simulink model "Racing_2019"  (R2017a)
settings: Solver=FixedStepDiscrete  StartTime=0.0  StopTime=Inf  FixedStep=1e-3  RelTol=1e-3  EnableMultiTasking=on
PostLoadFcn:
  | , if any(exist('dsrtsu_mdlpostloadfcn', 'file') == [2, 3, 6]), try dsrtsu_mdlpostloadfcn('Execute', bdroot); catch fprintf('Error in PostLoadFcn (dsrtsu_mdlpostloadfcn) for model "%s":\n %s\n', bdroot, lasterr); end, end,
undefined symbols (not defined in the file): Accu_Fans_Enable, Accu_Fans_ON, Accu_Fans_PWM, APPS_Bypass, APPS_Value, AUX_Error_Time, Batt_Temp_High_Threshold, Batt_Temp_Low_Threshold, BMS_Error_Time, BMS_Reset, BMS_Reset_Enable, BMS_Status_Bypass, Brake_Plausibility_Threshold, Brake_Threshold, Brakelight_Test, Braking_Torque, BSPD_State_Bypass, Buzzer, Buzzer_Silent, Buzzer_Test, Calibrate, CAN_Rx_FMEA_Enable, CAN_Status_FMEA_Enable, CAN_Tx_FMEA_Enable, Car_Reset, Car_Reset_Enable, Dash_Fan_PWM, DiscIntNeverNeededParam, DRS_Enable, DRS_PWM_OFF, DRS_PWM_ON, ED_Enable, ED_On, Eject_USB, Enable_Kill, Enable_LED_Test, Fans_Left_Enable, Fans_Left_ON, Fans_Left_PWM, Fans_Right_Enable, Fans_Right_ON, Fans_Right_PWM, I_MAX, IGBT_Temp_High_Threshold, IGBT_Temp_Low_Threshold, Inverter_CAN_Tx_Enable, Inverter_Frequency, KW_Max_Regen_Reset, KW_Max_Reset, LV_DCDC_Temp_High_Threshold, LV_DCDC_Temp_Low_Threshold, magnitude, Plausibility_Bypass, Power_Limiter_Killswitch, Power_Target_kW, Pump_Left_Enable, Pump_Left_ON, Pump_Right_Enable, Pump_Right_ON, Pump_Signal_Left ... (+13)
libraries: rtiusbflightreclib x206, simulink x153, rtican x52, powerlib_meascontrol x47, simulink_extras x17, rti1401lib_adc_type4 x6, rti1401lib_dio_type4 x3, rti1401lib_II_base x1
(part 6 of 23)

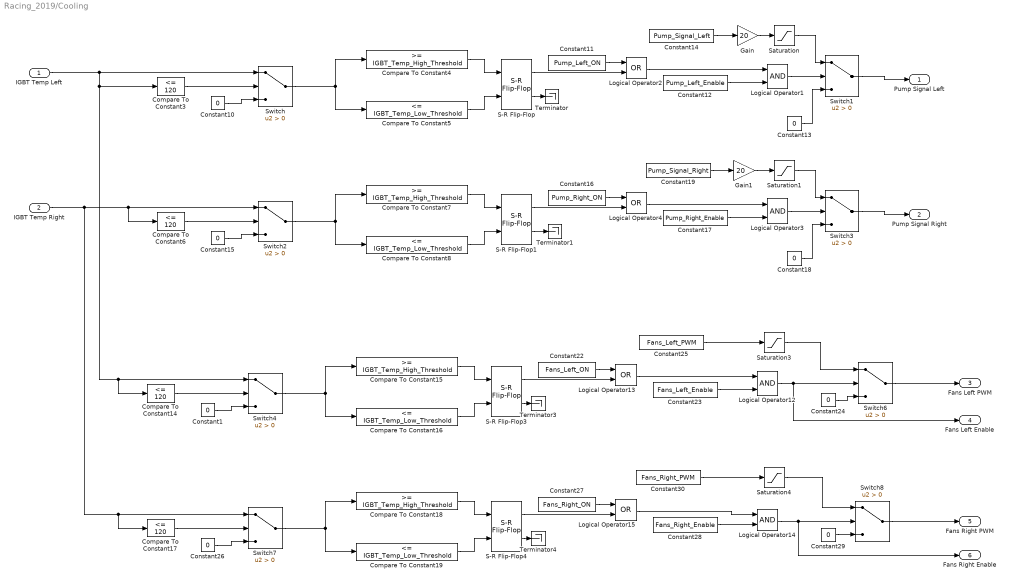
== system Racing_2019/Cooling ==
  IGBT Temp Left : Inport
  IGBT Temp Right : Inport  Port=2
  Compare To Constant{3,6,14,17} (4 alike) : simulink/Logic and Bit Operations/Compare To Constant  relop=<=  const=120  OutDataTypeStr=boolean
  Compare To Constant{4,7,15,18} (4 alike) : simulink/Logic and Bit Operations/Compare To Constant  relop=>=  const=IGBT_Temp_High_Threshold  OutDataTypeStr=boolean
  Compare To Constant{5,8,16,19} (4 alike) : simulink/Logic and Bit Operations/Compare To Constant  relop=<=  const=IGBT_Temp_Low_Threshold  OutDataTypeStr=boolean
  Constant{1,10,13,15,18,24,26,29} (8 alike) : Constant  Value=0
  Constant11 : Constant  Value=Pump_Left_ON
  Constant12 : Constant  Value=Pump_Left_Enable
  Constant14 : Constant  Value=Pump_Signal_Left  OutDataTypeStr=single
  Constant16 : Constant  Value=Pump_Right_ON
  Constant17 : Constant  Value=Pump_Right_Enable
  Constant19 : Constant  Value=Pump_Signal_Right  OutDataTypeStr=single
  Constant22 : Constant  Value=Fans_Left_ON
  Constant23 : Constant  Value=Fans_Left_Enable
  Constant25 : Constant  Value=Fans_Left_PWM  OutDataTypeStr=uint8
  Constant27 : Constant  Value=Fans_Right_ON
  Constant28 : Constant  Value=Fans_Right_Enable
  Constant30 : Constant  Value=Fans_Right_PWM  OutDataTypeStr=uint8
  Gain : Gain  Gain=20
  Gain1 : Gain  Gain=20
  Logical Operator{1,3,12,14} (4 alike) : Logic  AllPortsSameDT=off  OutDataTypeStr=boolean
  Logical Operator{2,4,13,15} (4 alike) : Logic  Operator=OR  AllPortsSameDT=off  OutDataTypeStr=boolean
  S-R Flip-Flop{,1,3..4} (4 alike) : simulink_extras/Flip Flops/S-R Flip-Flop  initial_condition=0
  Saturation{,1,3..4} (4 alike) : Saturate  UpperLimit=100  LowerLimit=0
  Switch{,1..4,6..8} (8 alike) : Switch  Criteria=u2 > Threshold
  Terminator{,1,3..4} (4 alike) : Terminator
  Pump Signal Left : Outport
  Pump Signal Right : Outport  Port=2
  "Fans Left PWM " : Outport  Port=3
  Fans Left Enable : Outport  Port=4
  Fans Right PWM : Outport  Port=5
  Fans Right Enable : Outport  Port=6
  wires:
  Compare To Constant3/1 -> Switch/2
  Compare To Constant4/1 -> S-R Flip-Flop/1
  Logical Operator2/1 -> Logical Operator1/1
  Constant11/1 -> Logical Operator2/1
  Logical Operator1/1 -> Switch1/2
  Constant12/1 -> Logical Operator1/2
  S-R Flip-Flop/2 -> Terminator/1
  Switch8/1 -> Fans Right PWM/1
  Constant14/1 -> Gain/1
  Switch3/1 -> Pump Signal Right/1
  Gain/1 -> Saturation/1
  S-R Flip-Flop/1 -> Logical Operator2/2
  Constant22/1 -> Logical Operator13/1
  Constant25/1 -> Saturation3/1
  Compare To Constant14/1 -> Switch4/2
  Compare To Constant15/1 -> S-R Flip-Flop3/1
  IGBT Temp Left/1 -> Switch/1, Compare To Constant3/1, Switch4/1, Compare To Constant14/1
  Logical Operator15/1 -> Logical Operator14/1
  Constant28/1 -> Logical Operator14/2
  Constant1/1 -> Switch4/3
  Constant26/1 -> Switch7/3
  Constant24/1 -> Switch6/3
  Compare To Constant19/1 -> S-R Flip-Flop4/2
  Compare To Constant17/1 -> Switch7/2
  Logical Operator13/1 -> Logical Operator12/1
  Constant30/1 -> Saturation4/1
  Saturation3/1 -> Switch6/1
  Switch4/1 -> Compare To Constant16/1, Compare To Constant15/1
  Compare To Constant16/1 -> S-R Flip-Flop3/2
  Switch7/1 -> Compare To Constant18/1, Compare To Constant19/1
  S-R Flip-Flop4/1 -> Logical Operator15/2
  Constant29/1 -> Switch8/3
  Constant23/1 -> Logical Operator12/2
  Compare To Constant18/1 -> S-R Flip-Flop4/1
  Logical Operator12/1 -> Fans Left Enable/1, Switch6/2
  S-R Flip-Flop3/1 -> Logical Operator13/2
  IGBT Temp Right/1 -> Switch7/1, Compare To Constant17/1, Switch2/1, Compare To Constant6/1
  Logical Operator14/1 -> Fans Right Enable/1, Switch8/2
  S-R Flip-Flop3/2 -> Terminator3/1
  Saturation4/1 -> Switch8/1
  S-R Flip-Flop4/2 -> Terminator4/1
  Constant27/1 -> Logical Operator15/1
  Gain1/1 -> Saturation1/1
  S-R Flip-Flop1/1 -> Logical Operator4/2
  Saturation1/1 -> Switch3/1
  Constant17/1 -> Logical Operator3/2
  S-R Flip-Flop1/2 -> Terminator1/1
  Constant19/1 -> Gain1/1
  Constant18/1 -> Switch3/3
  Compare To Constant8/1 -> S-R Flip-Flop1/2
  Compare To Constant6/1 -> Switch2/2
  Switch2/1 -> Compare To Constant7/1, Compare To Constant8/1
  Logical Operator3/1 -> Switch3/2
  Constant15/1 -> Switch2/3
  Compare To Constant7/1 -> S-R Flip-Flop1/1
  Logical Operator4/1 -> Logical Operator3/1
  Constant16/1 -> Logical Operator4/1
  Constant10/1 -> Switch/3
  Saturation/1 -> Switch1/1
  Constant13/1 -> Switch1/3
  Compare To Constant5/1 -> S-R Flip-Flop/2
  Switch/1 -> Compare To Constant5/1, Compare To Constant4/1
  Switch6/1 -> "Fans Left PWM "/1
  Switch1/1 -> Pump Signal Left/1

== system Racing_2019/DRS ==
  "APPS " : Inport
  "Brake " : Inport  Port=2
  Steering : Inport  Port=3
  Compare To Constant10 : simulink/Logic and Bit Operations/Compare To Constant  relop=>=  const=40  OutDataTypeStr=boolean
  Compare To Constant11 : simulink/Logic and Bit Operations/Compare To Constant  relop=<=  const=60  OutDataTypeStr=boolean
  Compare To Constant12 : simulink/Logic and Bit Operations/Compare To Constant  relop=<=  const=20  OutDataTypeStr=boolean
  Compare To Constant13 : simulink/Logic and Bit Operations/Compare To Constant  relop=>=  const=Brake_Threshold  OutDataTypeStr=boolean
  Compare To Constant9 : simulink/Logic and Bit Operations/Compare To Constant  relop=>=  const=800  OutDataTypeStr=boolean
  Constant20 : Constant  Value=DRS_PWM_ON
  Constant21 : Constant  Value=DRS_PWM_OFF
  Constant8 : Constant  Value=DRS_Enable
  Logical Operator10 : Logic  Operator=NOT  AllPortsSameDT=off  OutDataTypeStr=boolean
  Logical Operator11 : Logic  Operator=NOT  AllPortsSameDT=off  OutDataTypeStr=boolean
  Logical Operator5 : Logic  AllPortsSameDT=off  OutDataTypeStr=boolean
  Logical Operator6 : Logic  AllPortsSameDT=off  OutDataTypeStr=boolean
  Logical Operator7 : Logic  Operator=OR  AllPortsSameDT=off  OutDataTypeStr=boolean
  Logical Operator8 : Logic  Operator=OR  AllPortsSameDT=off  OutDataTypeStr=boolean
  Logical Operator9 : Logic  Operator=OR  Inputs=3  AllPortsSameDT=off  OutDataTypeStr=boolean
  S-R Flip-Flop2 : simulink_extras/Flip Flops/S-R Flip-Flop  initial_condition=0
  Saturation2 : Saturate  UpperLimit=100  LowerLimit=0
  Switch5 : Switch  Criteria=u2 > Threshold
  Terminator2 : Terminator
  DRS PWM : Outport
  wires:
  Compare To Constant11/1 -> Logical Operator5/2
  Compare To Constant10/1 -> Logical Operator5/1
  Compare To Constant9/1 -> Logical Operator6/1
  Logical Operator11/1 -> Logical Operator8/2
  Switch5/1 -> Saturation2/1
  S-R Flip-Flop2/2 -> Terminator2/1
  Constant20/1 -> Switch5/1
  Steering/1 -> Compare To Constant10/1, Compare To Constant11/1
  Compare To Constant12/1 -> Logical Operator9/2
  Logical Operator8/1 -> S-R Flip-Flop2/2
  Constant8/1 -> Logical Operator11/1, Logical Operator7/2
  Constant21/1 -> Switch5/3
  S-R Flip-Flop2/1 -> Switch5/2
  Logical Operator6/1 -> Logical Operator7/1
  Saturation2/1 -> DRS PWM/1
  "APPS "/1 -> Compare To Constant9/1, Compare To Constant12/1
  Logical Operator7/1 -> S-R Flip-Flop2/1
  Compare To Constant13/1 -> Logical Operator9/3
  Logical Operator5/1 -> Logical Operator6/2, Logical Operator10/1
  "Brake "/1 -> Compare To Constant13/1
  Logical Operator9/1 -> Logical Operator8/1
  Logical Operator10/1 -> Logical Operator9/1
